simulink model "ex2"  (R2021b)
settings: Solver=VariableStepAuto  StartTime=0.0  StopTime=20.0  RelTol=1e-3
settings Model: Creator=macbook  LastModifiedBy=macbook

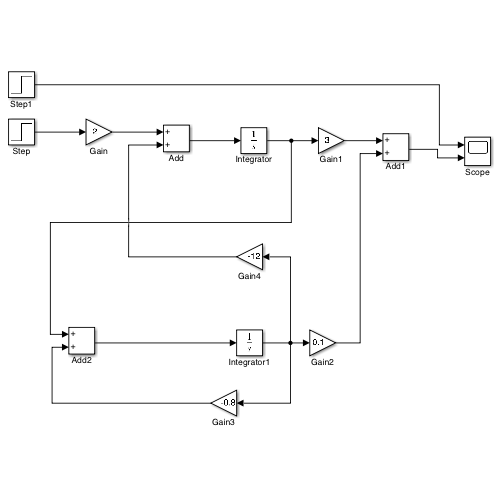
[thumbnail: Simulink's stored preview of the top-level diagram]
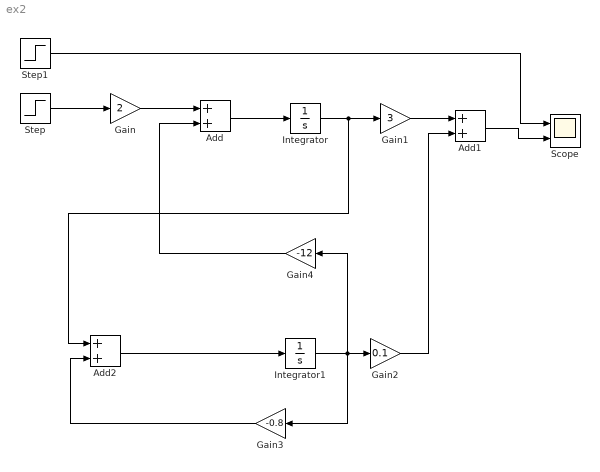
== system ex2 ==
  Add : Sum
  Add1 : Sum
  Add2 : Sum
  Gain : Gain  Gain=2
  Gain1 : Gain  Gain=3
  Gain2 : Gain  Gain=0.1
  Gain3 : Gain  Gain=-0.8
  Gain4 : Gain  Gain=-12
  Integrator : Integrator  InitialCondition=0.33
  Integrator1 : Integrator  InitialCondition=-0.5
  Scope : Scope  NumInputPorts=2
  Step : Step  After=0  SampleTime=0
  Step1 : Step  After=0  SampleTime=0
  wires:
  Step/1 -> Gain/1
  Gain/1 -> Add/1
  Add/1 -> Integrator/1
  Integrator/1 -> Gain1/1, Add2/1
  Gain1/1 -> Add1/1
  Gain2/1 -> Add1/2
  Integrator1/1 -> Gain4/1, Gain3/1, Gain2/1
  Add2/1 -> Integrator1/1
  Gain3/1 -> Add2/2
  Gain4/1 -> Add/2
  Add1/1 -> Scope/2
  Step1/1 -> Scope/1
